simulink model "model5"  (R2022a)
settings: Solver=VariableStepAuto  StartTime=0.0  StopTime=120  RelTol=1e-3
settings Model: Creator=tano-  LastModifiedBy=tano-

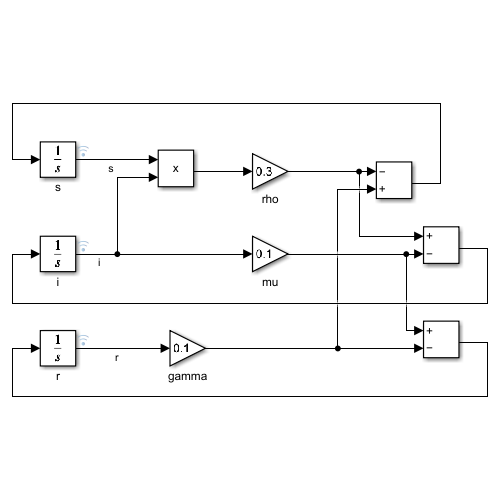
[thumbnail: Simulink's stored preview of the top-level diagram]
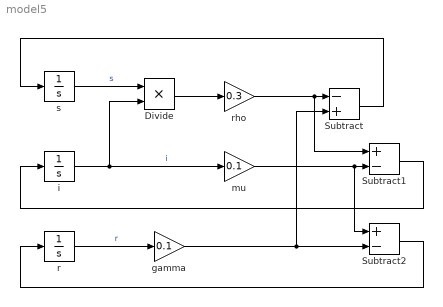
== system model5 ==
  Divide : Product  Inputs=**
  Subtract : Sum  Inputs=-+
  Subtract1 : Sum  Inputs=+-
  Subtract2 : Sum  Inputs=+-
  gamma : Gain  Gain=0.1
  i : Integrator  InitialCondition=0.0001
  mu : Gain  Gain=0.1
  r : Integrator
  rho : Gain  Gain=0.3
  s : Integrator  InitialCondition=0.9999
  wires:
  i/1 -> mu/1, Divide/2  "i"
  s/1 -> Divide/1  "s"
  r/1 -> gamma/1  "r"
  gamma/1 -> Subtract2/2, Subtract/2
  Divide/1 -> rho/1
  rho/1 -> Subtract1/1, Subtract/1
  Subtract/1 -> s/1
  mu/1 -> Subtract2/1, Subtract1/2
  Subtract1/1 -> i/1
  Subtract2/1 -> r/1
